simulink model "trajectory_block"  (R2013a)
settings: Solver=ode45  StartTime=0.0  StopTime=10.0  RelTol=1e-3
values from neighbouring files (symbols this model uses):
  ts = 0.01    [RUNCODE_Pointing_CntrlACT.m]
settings Model: Creator=Mike  LastModifiedBy=Mike

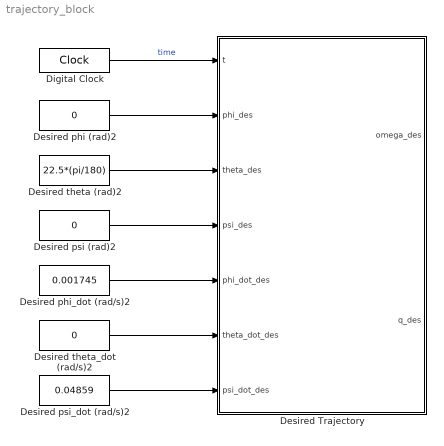
== system trajectory_block ==
  Desired Trajectory : MATLAB Function  TreatAsAtomicUnit=on
  Desired phi (rad)2 : Constant  Value=0
  Desired phi_dot (rad/s)2 : Constant  Value=0.001745
  Desired psi (rad)2 : Constant  Value=0
  Desired psi_dot (rad/s)2 : Constant  Value=0.04859
  Desired theta (rad)2 : Constant  Value=22.5*(pi/180)
  Desired theta_dot (rad/s)2 : Constant  Value=0
  Digital Clock : DigitalClock  SampleTime=ts
  wires:
  Digital Clock/1 -> Desired Trajectory/1(t)  "time"
  Desired theta (rad)2/1 -> Desired Trajectory/3(theta_des)
  Desired psi (rad)2/1 -> Desired Trajectory/4(psi_des)
  Desired theta_dot (rad/s)2/1 -> Desired Trajectory/6(theta_dot_des)
  Desired phi (rad)2/1 -> Desired Trajectory/2(phi_des)
  Desired phi_dot (rad/s)2/1 -> Desired Trajectory/5(phi_dot_des)
  Desired psi_dot (rad/s)2/1 -> Desired Trajectory/7(psi_dot_des)

== matlab function trajectory_block/Desired Trajectory ==
  data: t input; phi_des input; theta_des input; psi_des input; phi_dot_des input; theta_dot_des input; omega_des output; psi_dot_des input; q_des output
function [omega_des,q_des] = fcn(t,phi_des,theta_des,psi_des,phi_dot_des,theta_dot_des,psi_dot_des)

    %%  3-1-3 Attitude Matrix Parameters 
    s1 = sin(phi_des);
    s2 = sin(theta_des);
    s3 = sin(psi_des);
    c1 = cos(phi_des);
    c2 = cos(theta_des);
    c3 = cos(psi_des);

    A = [(c1*c3)-(s1*c2*s3), (c1*s3)+(s1*c2*c3), s1*s2;
         (-s1*c3)-(c1*c2*s3), (-s1*s3)+(c1*c2*c3) c1*s2;
          s2*s3,              -s2*c3,             c2;];

    %% Quaternion Parameters 
    q1_0 = sqrt((1/4)*(1+A(1,1)-A(2,2)-A(3,3)));
    q2_0 = sqrt((1/4)*(1+A(2,2)-A(1,1)-A(3,3)));
    q3_0 = sqrt((1/4)*(1+A(3,3)-A(1,1)-A(2,2)));
    q4_0 = sqrt((1/4)*(1+A(1,1)+A(2,2)+A(3,3)));
    q_0 = [q1_0 q2_0 q3_0 q4_0]';


    %% Desired Body Angular Velocity Trajectory 
    % Postion = velocity * time 
%     phi_des = phi_dot_des*t; %rad
  % theta = theta_dot*t; %rad --- THETA NOT CHANGING SINCE IT IS SPIN AXIS 
%     psi_des = psi_dot_des*t; %rad 

    ss1 = sin(phi_des);
    ss2 = sin(theta_des);
    ss3 = sin(psi_des);
    cc1 = cos(phi_des);
    cc2 = cos(theta_des);
    cc3 = cos(psi_des);

    % 3-1-3 Euler Angle Kinematic Differential Equation
    omega_des = inv((1/ss2)*[ss3, cc3, 0; ss2*cc3, -ss2*ss3, 0; -cc2*ss3, -cc2*cc3, ss2])*[phi_dot_des, theta_dot_des, psi_dot_des]';
    w1_des = omega_des(1,:);
    w2_des = omega_des(2,:);
    w3_des = omega_des(3,:);

    %% Kinematics Equation Propagation 
    % q_tilde(t + delta_t) = OMEGA_BAR[w_tilde(t)]q_tilde(t)
     % in seconds 
    zeta_t = (sin((1/2)*norm(omega_des)*t)*[w1_des, w2_des, w3_des]')/norm(omega_des);  

    % zeta cross parameters 
    zeta1 = zeta_t(1,:);
    zeta2 = zeta_t(2,:);
    zeta3 = zeta_t(3,:);

    % Cross product matrix for zeta 
    cross_zeta = [0       -zeta3   zeta2; 
                  zeta3    0      -zeta1; 
                 -zeta2    zeta1      0];

    % OMEGA_BAR[w_tilde(t)] parameters            
    row1col1 = cos((1/2)*norm(omega_des)*t)*eye(3)-cross_zeta;
    row1col2 = zeta_t;
    row2col1 = -zeta_t';
    row2col2 = cos((1/2)*norm(omega_des)*t);      

    OMEGA_BAR = [row1col1  row1col2; 
                 row2col1  row2col2]; 

    % Kinematics Equation    
    q_des = OMEGA_BAR*q_0;

    % Desired Quaternions
    q1_des = q_des(1,:)';
    q2_des = q_des(2,:)';
    q3_des = q_des(3,:)';
    q4_des = q_des(4,:)';
